simulink model "Customer"  (R2024b)
settings: Solver=VariableStepAuto  StartTime=0.0  StopTime=10.0  RelTol=1e-3
settings Model: Creator=CArias  LastModifiedBy=CArias

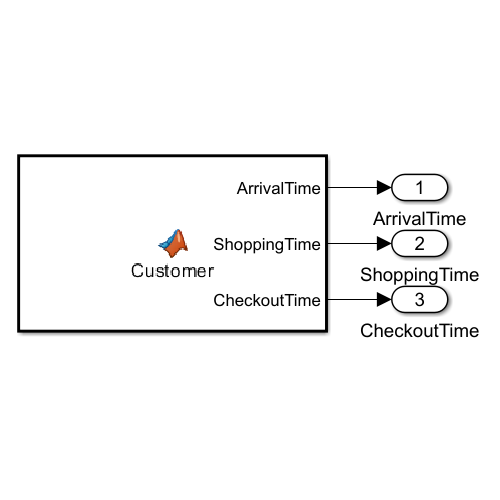
[thumbnail: Simulink's stored preview of the top-level diagram]
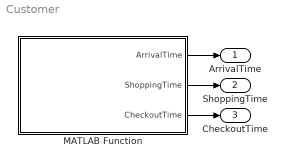
== system Customer ==
  MATLAB Function : MATLAB Function  TreatAsAtomicUnit=on
  ArrivalTime : Outport
  ShoppingTime : Outport  Port=2
  CheckoutTime : Outport  Port=3
  wires:
  MATLAB Function/1(ArrivalTime) -> ArrivalTime/1
  MATLAB Function/2(ShoppingTime) -> ShoppingTime/1
  MATLAB Function/3(CheckoutTime) -> CheckoutTime/1

== matlab function Customer/MATLAB Function ==
  data: ArrivalTime output; ShoppingTime output; CheckoutTime output
function [ArrivalTime, ShoppingTime, CheckoutTime] = Customer()

ArrivalTime = randi(10);
ShoppingTime = randi(7);
CheckoutTime = randi(4);
